simulink model "odeSolver"  (R2021b)
settings: Solver=VariableStepAuto  StartTime=0.0  StopTime=100  RelTol=1e-3
settings Model: Creator=ziyutian  LastModifiedBy=ziyutian

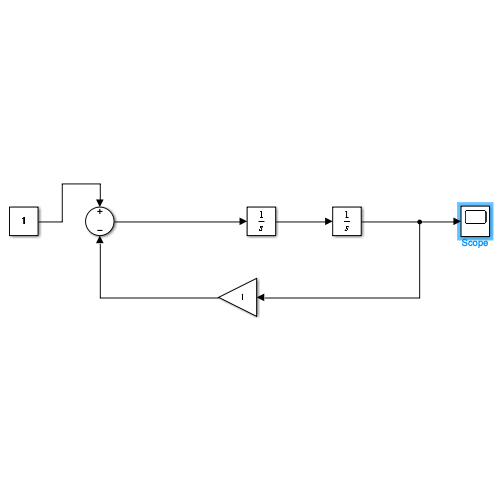
[thumbnail: Simulink's stored preview of the top-level diagram]
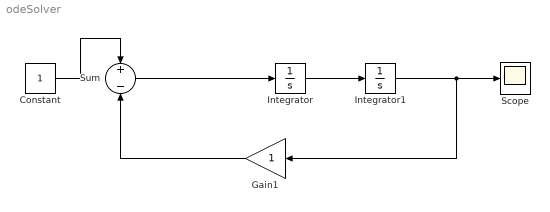
== system odeSolver ==
  Constant : Constant
  Gain1 : Gain
  Integrator : Integrator  InitialCondition=1
  Integrator1 : Integrator
  Scope : Scope
  Sum : Sum  Inputs=+-
  wires:
  Integrator/1 -> Integrator1/1
  Integrator1/1 -> Gain1/1, Scope/1
  Sum/1 -> Integrator/1
  Constant/1 -> Sum/1
  Gain1/1 -> Sum/2
